simulink model "MMMS_v3"  (R2024b)
settings: Solver=VariableStepAuto  StartTime=0.0  StopTime=60  FixedStep=0.001  RelTol=1e-3
InitFcn:
  | %rho_0t=[0.29;0.29;0.29]; %m
  | %V_0t=[-0.001;-0.001;0];%[-0.0005;-0.0005;0];
  | %w_t=[0;0;-0.002];
  | 
  | 
  | %rho_0t=[0.3;0.3;0.2]; %m
  | %V_0t=[-0.001;-0.001;0];%[-0.0005;-0.0005;0];
  | %w_t=[0;0;-0.001];
values from neighbouring files (symbols this model uses):
  Dt = 0.1    [main_EKF.m]
  Fake_Manip_grad = -0.2.*eye(7)    [Initiate_FQ.m]
  g_cm = zeros(4,4,n)    [Initiate_KUKA_inv.m]    (also in Main_MMMS.m; test_KUKA_elements.m)
  g_It00 = [eye(3) rho_It;0 0 0 1]    [main_EKF.m]
  iota0 = eye(6,6)    [Initiate_KUKA_inv.m]    (also in Main_MMMS.m; test_KUKA_elements.m)
  K_d = 10*[1.3*eye(3) zeros(3);zeros(3) 0.8*eye(3)]    [Initiate_FQ.m]    (also in Initiate_KUKA_inv.m = 5*[0.7*eye(3) zeros(3);zeros(3) 0.5*eye(3)]; MMMS_Initiate_FQ.m; Main_MMMS.m = 5*[0.7*eye(3) zeros(3);zeros(3) 0.5*eye(3)]; test_KUKA_elements.m = 50*[0.7*eye(3) zeros(3);zeros(3) 0.5*eye(3)])
  K_i = 5*[0.1*eye(3) zeros(3);zeros(3) 0.01*eye(3)]    [Initiate_FQ.m]    (also in Initiate_KUKA_inv.m = 5*[0.01*eye(3) zeros(3);zeros(3) 0.001*eye(3)]; MMMS_Initiate_FQ.m; Main_MMMS.m = 5*[0.01*eye(3) zeros(3);zeros(3) 0.001*eye(3)]; test_KUKA_elements.m = 50*[0.01*eye(3) zeros(3);zeros(3) 0.001*eye(3)])
  K_p = 100*[0.1 0 0 0 0 0;0 0.1 0 0 0 0; 0 0 0.1 0 0 0; 0 0 0 0.01 0 0 ... (first row only)    [Initiate_FQ.m]    (also in Initiate_KUKA_inv.m = 5*[0.1 0 0 0 0 0;0 0.1 0 0 0 0; 0 0 0.1 0 0 0; 0 0 0 0.01 0 ; MMMS_Initiate_FQ.m; Main_MMMS.m = 5*[0.1 0 0 0 0 0;0 0.1 0 0 0 0; 0 0 0.1 0 0 0; 0 0 0 0.01 0 ; test_KUKA_elements.m = 50*[0.1 0 0 0 0 0;0 0.1 0 0 0 0; 0 0 0.1 0 0 0; 0 0 0 0.01 0)
  K_w = 200*eye(7)    [Initiate_FQ.m]    (also in MMMS_Initiate_FQ.m)
  K_wd = 2*eye(7)    [Initiate_FQ.m]    (also in MMMS_Initiate_FQ.m)
  m = randn(s,total_time_steps,6)*chol(R)    [main_EKF.m]
  M0 = M_temp.M0.data(:,:,1)    [Initiate_FQ.m]    (also in MMMS_Initiate_FQ.m; test_KUKA_elements.m)
  m0 = robot.Bodies{1,n+1}.Mass    [Initiate_KUKA_inv.m]    (also in Main_MMMS.m; test_KUKA_elements.m)
  m0_frak = diag_M(1:6,1:6)    [Initiate_KUKA_inv.m]    (also in Main_MMMS.m; make_uncertain.m = diag_M_unc(1:6,1:6); test_KUKA_elements.m)
  M0m = M_temp.M0m.data(:,:,1)    [Initiate_FQ.m]    (also in MMMS_Initiate_FQ.m; test_KUKA_elements.m)
  m_diag = diag_M(7:end,7:end)    [Initiate_KUKA_inv.m]    (also in Main_MMMS.m; make_uncertain.m = diag_M_unc(7:end,7:end); test_KUKA_elements.m)
  M_t = (((Adjoint(g_It))'\M_t_body)/(Adjoint(g_It)))    [Initiate_FQ.m]    (also in Initiate_KUKA_inv.m = [eye(3)*mt zeros(3); zeros(3) eye(3)*80]; MMMS_Initiate_FQ.m; Main_MMMS.m = [eye(3)*mt zeros(3); zeros(3) eye(3)*80]; test_KUKA_elements.m = [eye(3)*mt zeros(3); zeros(3) eye(3)*80])
  M_t_body = [eye(3)*mt zeros(3); zeros(3) eye(3)*0.416667]    [Initiate_FQ.m]    (also in MMMS_Initiate_FQ.m)
  mm = zeros(1,n)    [Initiate_KUKA_inv.m]    (also in Main_MMMS.m; test_KUKA_elements.m)
  mu = P0    [Initiate_FQ.m]    (also in Initiate_KUKA_inv.m = zeros(6,1); MMMS_Initiate_FQ.m; Main_MMMS.m = zeros(6,1); make_uncertain.m = P0_unc)
  mu_t = inv((Adjoint(g_It))')*M_t_body*[V_It;w_t]    [Initiate_FQ.m]    (also in Initiate_KUKA_inv.m = M_t*[V_0t;w_t]; MMMS_Initiate_FQ.m; Main_MMMS.m = M_t*[V_0t;w_t]; make_uncertain.m = inv((Adjoint(g_It))')*M_t_body_unc*[V_It;w_t])
  noise_st = 0.000005    (= 5e-06)    [main_EKF.m]
  q_dot_m = [0;0;0;0;0;0;0]    [Initiate_FQ.m]    (also in Initiate_KUKA_inv.m; MMMS_Initiate_FQ.m; Main_MMMS.m; test_KUKA_elements.m = [0])
  q_m = [0.2;1.2;0.3;2.5;0.5;1.5;0.6]    [Initiate_FQ.m]    (also in Initiate_KUKA_inv.m = [0;0;0;0;0;0;0]; MMMS_Initiate_FQ.m = [0.2;0.2;0.3;0.5;0.5;0.5;0.6]; Main_MMMS.m = [0;0;0;0;0;0;0]; test_KUKA_elements.m = [0.2;1.2;0.3;1.8;0.5;1.3;0.6])
  rho_It = [0;0;1.7]    [Initiate_FQ.m]    (also in MMMS_Initiate_FQ.m)
  s = RandStream.create('mrg32k3a','NumStreams',1)    [main_EKF.m]
  sc_size = 1    [Initiate_KUKA_inv.m]    (also in Main_MMMS.m; test_KUKA_elements.m)
  V_It = [0.0005;0.0005;0]    [Initiate_FQ.m]    (also in MMMS_Initiate_FQ.m = [0.001;0.001;0])
  Xi_m_matrix = zeros(6*n,n)    [Initiate_KUKA_inv.m]    (also in Main_MMMS.m)
undefined symbols (not defined in the file or in its folder): g_cm0, I0, Im, Mm, X, Xi_m, Y, Z
libraries: nesl_utility x314, sm_lib x231, robotcorelib x30, simulink x12
(part 10 of 13)

== system MMMS_v3/MMS4/joint//link2/iiwa_link_2 ==
  Inertia : sm_lib/Body Elements/Inertia  InertiaType=Custom  Mass=mm(5)  MassUnits=kg  CenterOfMass=[0, 0, 0]  CenterOfMassUnits=m  MomentsOfInertia=[Im(1,1,5) Im(2,2,5) Im(3,3,5)]  MomentsOfInertiaUnits=kg*m^2  ProductsOfInertia=[Im(3,2,5) Im(3,1,5) Im(2,1,5)]  ProductsOfInertiaUnits=kg*m^2  GraphicType=None  MarkerShape=Inertia  MarkerSize=20  GraphicVisPropType=SimpleVisualProperties  GraphicDiffuseColor=[0.5 0.5 0.5]  GraphicOpacity=1.0  GraphicSpecularColor=[0.5 0.5 0.5 1.0]  GraphicAmbientColor=[0.15 0.15 0.15 1.0]  GraphicEmissiveColor=[0.0 0.0 0.0 1.0]  GraphicShininess=75
  Visual : sm_lib/Body Elements/File Solid  ExtGeomFileName=iiwa_description/meshes/iiwa7/visual/link_2.stl  UnitType=Custom  ExtGeomFileUnits=m  StepReaderType=HEX  ExportConvexHullGeometry=off  InertiaType=Custom  BasedOnType=DensityFromFile  Density=1000  DensityUnits=kg/m^3  Mass=0  MassUnits=kg  CenterOfMass=[0, 0, 0]  CenterOfMassUnits=m  MomentsOfInertia=[0, 0, 0]  MomentsOfInertiaUnits=kg*m^2  ProductsOfInertia=[0, 0, 0]  ProductsOfInertiaUnits=kg*m^2  GraphicType=FromGeometry  MarkerShape=Sphere  MarkerSize=10  GraphicVisPropType=SimpleVisualProperties  GraphicDiffuseColor=[1, 0.423529411765, 0.0392156862745]  GraphicOpacity=1  GraphicSpecularColor=[0.5 0.5 0.5 1.0]  GraphicAmbientColor=[0.15 0.15 0.15 1.0]  GraphicEmissiveColor=[0.0 0.0 0.0 1.0]  GraphicShininess=75  DoExposeReferenceFrame=on  SerializedFrames=<Frames/>
  VisualOriginTransform : sm_lib/Frames and Transforms/Rigid Transform  RotationMethod=RotationSequence  FollAlignAxisA=+X  BaseAlignAxisA=+Y  FollAlignAxisB=+Y  BaseAlignAxisB=+Z  RotationStandardAxis=+Z  RotationAngle=0.0  RotationAngleUnits=deg  RotationArbitraryAxis=[0 0 1]  RotationSequenceAxes=BaseAxes  RotationSequence=XYZ  RotationSequenceAngles=[0, 0, 0]  RotationSequenceAnglesUnits=rad  RotationMatrix=[1 0 0; 0 1 0; 0 0 1]  Quaternion=[1 0 0 0]  TranslationMethod=Cartesian  TranslationCartesianOffset=[0, 0, 0]  TranslationCartesianOffsetUnits=m  TranslationStandardAxis=+Z  TranslationStandardOffset=0  TranslationStandardOffsetUnits=m  TranslationROffset=0  TranslationROffsetUnits=m  TranslationThetaOffset=0  TranslationThetaOffsetUnits=deg  TranslationZOffset=0  TranslationZOffsetUnits=m
  iiwa_joint_3_OriginTransform : sm_lib/Frames and Transforms/Rigid Transform  RotationMethod=RotationMatrix  FollAlignAxisA=+X  BaseAlignAxisA=+Y  FollAlignAxisB=+Y  BaseAlignAxisB=+Z  RotationStandardAxis=+Z  RotationAngle=0.0  RotationAngleUnits=deg  RotationArbitraryAxis=[0 0 1]  RotationSequenceAxes=BaseAxes  RotationSequence=XYZ  RotationSequenceAngles=[1.57079632679, 0, 3.14159265359]  RotationSequenceAnglesUnits=rad  RotationMatrix=g_cm(1:3,1:3,5)  Quaternion=[1 0 0 0]  TranslationMethod=Cartesian  TranslationCartesianOffset=g_cm(1:3,4,5)'  TranslationCartesianOffsetUnits=m  TranslationStandardAxis=+Z  TranslationStandardOffset=0  TranslationStandardOffsetUnits=m  TranslationROffset=0  TranslationROffsetUnits=m  TranslationThetaOffset=0  TranslationThetaOffsetUnits=deg  TranslationZOffset=0  TranslationZOffsetUnits=m
  F : PMIOPort  Side=Left
  F1 : PMIOPort  Port=2  Side=Right
  connections:
  iiwa_joint_3_OriginTransform/LConn1 -- F1/RConn1
  F/RConn1 -- iiwa_joint_3_OriginTransform/RConn1 -- Inertia/RConn1 -- VisualOriginTransform/LConn1
  Visual/RConn1 -- VisualOriginTransform/RConn1

== system MMMS_v3/MMS4/joint//link3/iiwa_link_3 ==
  Inertia : sm_lib/Body Elements/Inertia  InertiaType=Custom  Mass=mm(4)  MassUnits=kg  CenterOfMass=[0, 0, 0]  CenterOfMassUnits=m  MomentsOfInertia=[Im(1,1,4) Im(2,2,4) Im(3,3,4)]  MomentsOfInertiaUnits=kg*m^2  ProductsOfInertia=[Im(3,2,4) Im(3,1,4) Im(2,1,4)]  ProductsOfInertiaUnits=kg*m^2  GraphicType=None  MarkerShape=Inertia  MarkerSize=20  GraphicVisPropType=SimpleVisualProperties  GraphicDiffuseColor=[0.5 0.5 0.5]  GraphicOpacity=1.0  GraphicSpecularColor=[0.5 0.5 0.5 1.0]  GraphicAmbientColor=[0.15 0.15 0.15 1.0]  GraphicEmissiveColor=[0.0 0.0 0.0 1.0]  GraphicShininess=75
  Visual : sm_lib/Body Elements/File Solid  ExtGeomFileName=iiwa_description/meshes/iiwa7/visual/link_3.stl  UnitType=Custom  ExtGeomFileUnits=m  StepReaderType=HEX  ExportConvexHullGeometry=off  InertiaType=Custom  BasedOnType=DensityFromFile  Density=1000  DensityUnits=kg/m^3  Mass=0  MassUnits=kg  CenterOfMass=[0, 0, 0]  CenterOfMassUnits=m  MomentsOfInertia=[0, 0, 0]  MomentsOfInertiaUnits=kg*m^2  ProductsOfInertia=[0, 0, 0]  ProductsOfInertiaUnits=kg*m^2  GraphicType=FromGeometry  MarkerShape=Sphere  MarkerSize=10  GraphicVisPropType=SimpleVisualProperties  GraphicDiffuseColor=[1, 0.423529411765, 0.0392156862745]  GraphicOpacity=1  GraphicSpecularColor=[0.5 0.5 0.5 1.0]  GraphicAmbientColor=[0.15 0.15 0.15 1.0]  GraphicEmissiveColor=[0.0 0.0 0.0 1.0]  GraphicShininess=75  DoExposeReferenceFrame=on  SerializedFrames=<Frames/>
  VisualOriginTransform : sm_lib/Frames and Transforms/Rigid Transform  RotationMethod=RotationSequence  FollAlignAxisA=+X  BaseAlignAxisA=+Y  FollAlignAxisB=+Y  BaseAlignAxisB=+Z  RotationStandardAxis=+Z  RotationAngle=0.0  RotationAngleUnits=deg  RotationArbitraryAxis=[0 0 1]  RotationSequenceAxes=BaseAxes  RotationSequence=XYZ  RotationSequenceAngles=[0, 0, 0]  RotationSequenceAnglesUnits=rad  RotationMatrix=[1 0 0; 0 1 0; 0 0 1]  Quaternion=[1 0 0 0]  TranslationMethod=Cartesian  TranslationCartesianOffset=[0, 0, -0.026]  TranslationCartesianOffsetUnits=m  TranslationStandardAxis=+Z  TranslationStandardOffset=0  TranslationStandardOffsetUnits=m  TranslationROffset=0  TranslationROffsetUnits=m  TranslationThetaOffset=0  TranslationThetaOffsetUnits=deg  TranslationZOffset=0  TranslationZOffsetUnits=m
  iiwa_joint_4_OriginTransform : sm_lib/Frames and Transforms/Rigid Transform  RotationMethod=RotationMatrix  FollAlignAxisA=+X  BaseAlignAxisA=+Y  FollAlignAxisB=+Y  BaseAlignAxisB=+Z  RotationStandardAxis=+Z  RotationAngle=0.0  RotationAngleUnits=deg  RotationArbitraryAxis=[0 0 1]  RotationSequenceAxes=BaseAxes  RotationSequence=XYZ  RotationSequenceAngles=[1.57079632679, 0, 0]  RotationSequenceAnglesUnits=rad  RotationMatrix=g_cm(1:3,1:3,4)  Quaternion=[1 0 0 0]  TranslationMethod=Cartesian  TranslationCartesianOffset=g_cm(1:3,4,4)'  TranslationCartesianOffsetUnits=m  TranslationStandardAxis=+Z  TranslationStandardOffset=0  TranslationStandardOffsetUnits=m  TranslationROffset=0  TranslationROffsetUnits=m  TranslationThetaOffset=0  TranslationThetaOffsetUnits=deg  TranslationZOffset=0  TranslationZOffsetUnits=m
  F : PMIOPort  Side=Left
  F1 : PMIOPort  Port=2  Side=Right
  connections:
  iiwa_joint_4_OriginTransform/LConn1 -- F1/RConn1
  Visual/RConn1 -- VisualOriginTransform/RConn1
  F/RConn1 -- Inertia/RConn1 -- iiwa_joint_4_OriginTransform/RConn1 -- VisualOriginTransform/LConn1

== system MMMS_v3/MMS4/joint//link4/iiwa_link_4 ==
  Inertia : sm_lib/Body Elements/Inertia  InertiaType=Custom  Mass=mm(3)  MassUnits=kg  CenterOfMass=[0, 0, 0]  CenterOfMassUnits=m  MomentsOfInertia=[Im(1,1,3) Im(2,2,3) Im(3,3,3)]  MomentsOfInertiaUnits=kg*m^2  ProductsOfInertia=[Im(3,2,3) Im(3,1,3) Im(2,1,3)]  ProductsOfInertiaUnits=kg*m^2  GraphicType=None  MarkerShape=Inertia  MarkerSize=20  GraphicVisPropType=SimpleVisualProperties  GraphicDiffuseColor=[0.5 0.5 0.5]  GraphicOpacity=1.0  GraphicSpecularColor=[0.5 0.5 0.5 1.0]  GraphicAmbientColor=[0.15 0.15 0.15 1.0]  GraphicEmissiveColor=[0.0 0.0 0.0 1.0]  GraphicShininess=75
  Visual : sm_lib/Body Elements/File Solid  ExtGeomFileName=iiwa_description/meshes/iiwa7/visual/link_4.stl  UnitType=Custom  ExtGeomFileUnits=m  StepReaderType=HEX  ExportConvexHullGeometry=off  InertiaType=Custom  BasedOnType=DensityFromFile  Density=1000  DensityUnits=kg/m^3  Mass=0  MassUnits=kg  CenterOfMass=[0, 0, 0]  CenterOfMassUnits=m  MomentsOfInertia=[0, 0, 0]  MomentsOfInertiaUnits=kg*m^2  ProductsOfInertia=[0, 0, 0]  ProductsOfInertiaUnits=kg*m^2  GraphicType=FromGeometry  MarkerShape=Sphere  MarkerSize=10  GraphicVisPropType=SimpleVisualProperties  GraphicDiffuseColor=[1, 0.423529411765, 0.0392156862745]  GraphicOpacity=1  GraphicSpecularColor=[0.5 0.5 0.5 1.0]  GraphicAmbientColor=[0.15 0.15 0.15 1.0]  GraphicEmissiveColor=[0.0 0.0 0.0 1.0]  GraphicShininess=75  DoExposeReferenceFrame=on  SerializedFrames=<Frames/>
  VisualOriginTransform : sm_lib/Frames and Transforms/Rigid Transform  RotationMethod=RotationSequence  FollAlignAxisA=+X  BaseAlignAxisA=+Y  FollAlignAxisB=+Y  BaseAlignAxisB=+Z  RotationStandardAxis=+Z  RotationAngle=0.0  RotationAngleUnits=deg  RotationArbitraryAxis=[0 0 1]  RotationSequenceAxes=BaseAxes  RotationSequence=XYZ  RotationSequenceAngles=[0, 0, 0]  RotationSequenceAnglesUnits=rad  RotationMatrix=[1 0 0; 0 1 0; 0 0 1]  Quaternion=[1 0 0 0]  TranslationMethod=Cartesian  TranslationCartesianOffset=[0, 0, 0]  TranslationCartesianOffsetUnits=m  TranslationStandardAxis=+Z  TranslationStandardOffset=0  TranslationStandardOffsetUnits=m  TranslationROffset=0  TranslationROffsetUnits=m  TranslationThetaOffset=0  TranslationThetaOffsetUnits=deg  TranslationZOffset=0  TranslationZOffsetUnits=m
  iiwa_joint_5_OriginTransform : sm_lib/Frames and Transforms/Rigid Transform  RotationMethod=RotationMatrix  FollAlignAxisA=+X  BaseAlignAxisA=+Y  FollAlignAxisB=+Y  BaseAlignAxisB=+Z  RotationStandardAxis=+Z  RotationAngle=0.0  RotationAngleUnits=deg  RotationArbitraryAxis=[0 0 1]  RotationSequenceAxes=BaseAxes  RotationSequence=XYZ  RotationSequenceAngles=[-1.57079632679, 3.14159265359, 0]  RotationSequenceAnglesUnits=rad  RotationMatrix=g_cm(1:3,1:3,3)  Quaternion=[1 0 0 0]  TranslationMethod=Cartesian  TranslationCartesianOffset=g_cm(1:3,4,3)'  TranslationCartesianOffsetUnits=m  TranslationStandardAxis=+Z  TranslationStandardOffset=0  TranslationStandardOffsetUnits=m  TranslationROffset=0  TranslationROffsetUnits=m  TranslationThetaOffset=0  TranslationThetaOffsetUnits=deg  TranslationZOffset=0  TranslationZOffsetUnits=m
  F : PMIOPort  Side=Left
  F1 : PMIOPort  Port=2  Side=Right
  connections:
  iiwa_joint_5_OriginTransform/LConn1 -- F1/RConn1
  F/RConn1 -- iiwa_joint_5_OriginTransform/RConn1 -- Inertia/RConn1 -- VisualOriginTransform/LConn1
  Visual/RConn1 -- VisualOriginTransform/RConn1

== system MMMS_v3/MMS4/joint//link5/iiwa_link_5 ==
  Inertia : sm_lib/Body Elements/Inertia  InertiaType=Custom  Mass=mm(2)  MassUnits=kg  CenterOfMass=[0, 0, 0]  CenterOfMassUnits=m  MomentsOfInertia=[Im(1,1,2) Im(2,2,2) Im(3,3,2)]  MomentsOfInertiaUnits=kg*m^2  ProductsOfInertia=[Im(3,2,2) Im(3,1,2) Im(2,1,2)]  ProductsOfInertiaUnits=kg*m^2  GraphicType=None  MarkerShape=Inertia  MarkerSize=20  GraphicVisPropType=SimpleVisualProperties  GraphicDiffuseColor=[0.5 0.5 0.5]  GraphicOpacity=1.0  GraphicSpecularColor=[0.5 0.5 0.5 1.0]  GraphicAmbientColor=[0.15 0.15 0.15 1.0]  GraphicEmissiveColor=[0.0 0.0 0.0 1.0]  GraphicShininess=75
  Visual : sm_lib/Body Elements/File Solid  ExtGeomFileName=iiwa_description/meshes/iiwa7/visual/link_5.stl  UnitType=Custom  ExtGeomFileUnits=m  StepReaderType=HEX  ExportConvexHullGeometry=off  InertiaType=Custom  BasedOnType=DensityFromFile  Density=1000  DensityUnits=kg/m^3  Mass=0  MassUnits=kg  CenterOfMass=[0, 0, 0]  CenterOfMassUnits=m  MomentsOfInertia=[0, 0, 0]  MomentsOfInertiaUnits=kg*m^2  ProductsOfInertia=[0, 0, 0]  ProductsOfInertiaUnits=kg*m^2  GraphicType=FromGeometry  MarkerShape=Sphere  MarkerSize=10  GraphicVisPropType=SimpleVisualProperties  GraphicDiffuseColor=[1, 0.423529411765, 0.0392156862745]  GraphicOpacity=1  GraphicSpecularColor=[0.5 0.5 0.5 1.0]  GraphicAmbientColor=[0.15 0.15 0.15 1.0]  GraphicEmissiveColor=[0.0 0.0 0.0 1.0]  GraphicShininess=75  DoExposeReferenceFrame=on  SerializedFrames=<Frames/>
  VisualOriginTransform : sm_lib/Frames and Transforms/Rigid Transform  RotationMethod=RotationSequence  FollAlignAxisA=+X  BaseAlignAxisA=+Y  FollAlignAxisB=+Y  BaseAlignAxisB=+Z  RotationStandardAxis=+Z  RotationAngle=0.0  RotationAngleUnits=deg  RotationArbitraryAxis=[0 0 1]  RotationSequenceAxes=BaseAxes  RotationSequence=XYZ  RotationSequenceAngles=[0, 0, 0]  RotationSequenceAnglesUnits=rad  RotationMatrix=[1 0 0; 0 1 0; 0 0 1]  Quaternion=[1 0 0 0]  TranslationMethod=Cartesian  TranslationCartesianOffset=[0, 0, -0.026]  TranslationCartesianOffsetUnits=m  TranslationStandardAxis=+Z  TranslationStandardOffset=0  TranslationStandardOffsetUnits=m  TranslationROffset=0  TranslationROffsetUnits=m  TranslationThetaOffset=0  TranslationThetaOffsetUnits=deg  TranslationZOffset=0  TranslationZOffsetUnits=m
  iiwa_joint_6_OriginTransform : sm_lib/Frames and Transforms/Rigid Transform  Commented=on  RotationMethod=RotationSequence  FollAlignAxisA=+X  BaseAlignAxisA=+Y  FollAlignAxisB=+Y  BaseAlignAxisB=+Z  RotationStandardAxis=+Z  RotationAngle=0.0  RotationAngleUnits=deg  RotationArbitraryAxis=[0 0 1]  RotationSequenceAxes=BaseAxes  RotationSequence=XYZ  RotationSequenceAngles=[1.57079632679, 0, 0]  RotationSequenceAnglesUnits=rad  RotationMatrix=[1 0 0; 0 1 0; 0 0 1]  Quaternion=[1 0 0 0]  TranslationMethod=Cartesian  TranslationCartesianOffset=[0, 0.0607 , 0.19]  TranslationCartesianOffsetUnits=m  TranslationStandardAxis=+Z  TranslationStandardOffset=0  TranslationStandardOffsetUnits=m  TranslationROffset=0  TranslationROffsetUnits=m  TranslationThetaOffset=0  TranslationThetaOffsetUnits=deg  TranslationZOffset=0  TranslationZOffsetUnits=m
  iiwa_joint_6_OriginTransform1 : sm_lib/Frames and Transforms/Rigid Transform  RotationMethod=RotationMatrix  FollAlignAxisA=+X  BaseAlignAxisA=+Y  FollAlignAxisB=+Y  BaseAlignAxisB=+Z  RotationStandardAxis=+Z  RotationAngle=0.0  RotationAngleUnits=deg  RotationArbitraryAxis=[0 0 1]  RotationSequenceAxes=BaseAxes  RotationSequence=XYZ  RotationSequenceAngles=[1.57079632679, 0, 0]  RotationSequenceAnglesUnits=rad  RotationMatrix=g_cm(1:3,1:3,2)  Quaternion=[1 0 0 0]  TranslationMethod=Cartesian  TranslationCartesianOffset=g_cm(1:3,4,2)'  TranslationCartesianOffsetUnits=m  TranslationStandardAxis=+Z  TranslationStandardOffset=0  TranslationStandardOffsetUnits=m  TranslationROffset=0  TranslationROffsetUnits=m  TranslationThetaOffset=0  TranslationThetaOffsetUnits=deg  TranslationZOffset=0  TranslationZOffsetUnits=m
  F : PMIOPort  Side=Left
  F1 : PMIOPort  Port=2  Side=Right
  connections:
  iiwa_joint_6_OriginTransform1/LConn1 -- F1/RConn1
  F/RConn1 -- VisualOriginTransform/LConn1 -- Inertia/RConn1 -- iiwa_joint_6_OriginTransform1/RConn1
  Visual/RConn1 -- VisualOriginTransform/RConn1

== system MMMS_v3/MMS4/joint//link6/iiwa_link_6 ==
  Inertia : sm_lib/Body Elements/Inertia  InertiaType=Custom  Mass=mm(1)  MassUnits=kg  CenterOfMass=[0, 0, 0]  CenterOfMassUnits=m  MomentsOfInertia=[Im(1,1,1) Im(2,2,1) Im(3,3,1)]  MomentsOfInertiaUnits=kg*m^2  ProductsOfInertia=[Im(3,2,1) Im(3,1,1) Im(2,1,1)]  ProductsOfInertiaUnits=kg*m^2  GraphicType=None  MarkerShape=Inertia  MarkerSize=20  GraphicVisPropType=SimpleVisualProperties  GraphicDiffuseColor=[0.5 0.5 0.5]  GraphicOpacity=1.0  GraphicSpecularColor=[0.5 0.5 0.5 1.0]  GraphicAmbientColor=[0.15 0.15 0.15 1.0]  GraphicEmissiveColor=[0.0 0.0 0.0 1.0]  GraphicShininess=75
  Visual : sm_lib/Body Elements/File Solid  ExtGeomFileName=iiwa_description/meshes/iiwa7/visual/link_6.stl  UnitType=Custom  ExtGeomFileUnits=m  StepReaderType=HEX  ExportConvexHullGeometry=off  InertiaType=Custom  BasedOnType=DensityFromFile  Density=1000  DensityUnits=kg/m^3  Mass=0  MassUnits=kg  CenterOfMass=[0, 0, 0]  CenterOfMassUnits=m  MomentsOfInertia=[0, 0, 0]  MomentsOfInertiaUnits=kg*m^2  ProductsOfInertia=[0, 0, 0]  ProductsOfInertiaUnits=kg*m^2  GraphicType=FromGeometry  MarkerShape=Sphere  MarkerSize=10  GraphicVisPropType=SimpleVisualProperties  GraphicDiffuseColor=[1, 0.423529411765, 0.0392156862745]  GraphicOpacity=1  GraphicSpecularColor=[0.5 0.5 0.5 1.0]  GraphicAmbientColor=[0.15 0.15 0.15 1.0]  GraphicEmissiveColor=[0.0 0.0 0.0 1.0]  GraphicShininess=75  DoExposeReferenceFrame=on  SerializedFrames=<Frames/>
  VisualOriginTransform : sm_lib/Frames and Transforms/Rigid Transform  RotationMethod=RotationSequence  FollAlignAxisA=+X  BaseAlignAxisA=+Y  FollAlignAxisB=+Y  BaseAlignAxisB=+Z  RotationStandardAxis=+Z  RotationAngle=0.0  RotationAngleUnits=deg  RotationArbitraryAxis=[0 0 1]  RotationSequenceAxes=BaseAxes  RotationSequence=XYZ  RotationSequenceAngles=[0, 0, 0]  RotationSequenceAnglesUnits=rad  RotationMatrix=[1 0 0; 0 1 0; 0 0 1]  Quaternion=[1 0 0 0]  TranslationMethod=Cartesian  TranslationCartesianOffset=[0, 0, 0.0607 ]  TranslationCartesianOffsetUnits=m  TranslationStandardAxis=+Z  TranslationStandardOffset=0  TranslationStandardOffsetUnits=m  TranslationROffset=0  TranslationROffsetUnits=m  TranslationThetaOffset=0  TranslationThetaOffsetUnits=deg  TranslationZOffset=0  TranslationZOffsetUnits=m
  iiwa_joint_7_OriginTransform : sm_lib/Frames and Transforms/Rigid Transform  RotationMethod=RotationMatrix  FollAlignAxisA=+X  BaseAlignAxisA=+Y  FollAlignAxisB=+Y  BaseAlignAxisB=+Z  RotationStandardAxis=+Z  RotationAngle=0.0  RotationAngleUnits=deg  RotationArbitraryAxis=[0 0 1]  RotationSequenceAxes=BaseAxes  RotationSequence=XYZ  RotationSequenceAngles=[-1.57079632679, 3.14159265359, 0]  RotationSequenceAnglesUnits=rad  RotationMatrix=g_cm(1:3,1:3,1)  Quaternion=[1 0 0 0]  TranslationMethod=Cartesian  TranslationCartesianOffset=g_cm(1:3,4,1)'  TranslationCartesianOffsetUnits=m  TranslationStandardAxis=+Z  TranslationStandardOffset=0  TranslationStandardOffsetUnits=m  TranslationROffset=0  TranslationROffsetUnits=m  TranslationThetaOffset=0  TranslationThetaOffsetUnits=deg  TranslationZOffset=0  TranslationZOffsetUnits=m
  F : PMIOPort  Side=Left
  F1 : PMIOPort  Port=2  Side=Right
  connections:
  iiwa_joint_7_OriginTransform/LConn1 -- F1/RConn1
  Visual/RConn1 -- VisualOriginTransform/RConn1
  VisualOriginTransform/LConn1 -- F/RConn1 -- Inertia/RConn1 -- iiwa_joint_7_OriginTransform/RConn1

== system MMMS_v3/MMS4/joint//link7/iiwa_link_7 ==
  Inertia : sm_lib/Body Elements/Inertia  InertiaType=Custom  Mass=m0  MassUnits=kg  CenterOfMass=[0, 0, 0]  CenterOfMassUnits=m  MomentsOfInertia=[I0(1,1) I0(2,2) I0(3,3)]  MomentsOfInertiaUnits=kg*m^2  ProductsOfInertia=[I0(3,2) I0(3,1) I0(2,1)]  ProductsOfInertiaUnits=kg*m^2  GraphicType=None  MarkerShape=Inertia  MarkerSize=20  GraphicVisPropType=SimpleVisualProperties  GraphicDiffuseColor=[0.5 0.5 0.5]  GraphicOpacity=1.0  GraphicSpecularColor=[0.5 0.5 0.5 1.0]  GraphicAmbientColor=[0.15 0.15 0.15 1.0]  GraphicEmissiveColor=[0.0 0.0 0.0 1.0]  GraphicShininess=75
  Visual : sm_lib/Body Elements/File Solid  ExtGeomFileName=iiwa_description/meshes/iiwa7/visual/link_7.stl  UnitType=Custom  ExtGeomFileUnits=m  StepReaderType=HEX  ExportConvexHullGeometry=off  InertiaType=Custom  BasedOnType=DensityFromFile  Density=1000  DensityUnits=kg/m^3  Mass=0  MassUnits=kg  CenterOfMass=[0, 0, 0]  CenterOfMassUnits=m  MomentsOfInertia=[0, 0, 0]  MomentsOfInertiaUnits=kg*m^2  ProductsOfInertia=[0, 0, 0]  ProductsOfInertiaUnits=kg*m^2  GraphicType=FromGeometry  MarkerShape=Sphere  MarkerSize=10  GraphicVisPropType=SimpleVisualProperties  GraphicDiffuseColor=[0.4, 0.4, 0.4]  GraphicOpacity=1  GraphicSpecularColor=[0.5 0.5 0.5 1.0]  GraphicAmbientColor=[0.15 0.15 0.15 1.0]  GraphicEmissiveColor=[0.0 0.0 0.0 1.0]  GraphicShininess=75  DoExposeReferenceFrame=on  SerializedFrames=<Frames/>
  VisualOriginTransform : sm_lib/Frames and Transforms/Rigid Transform  RotationMethod=RotationSequence  FollAlignAxisA=+X  BaseAlignAxisA=+Y  FollAlignAxisB=+Y  BaseAlignAxisB=+Z  RotationStandardAxis=+Z  RotationAngle=0.0  RotationAngleUnits=deg  RotationArbitraryAxis=[0 0 1]  RotationSequenceAxes=BaseAxes  RotationSequence=XYZ  RotationSequenceAngles=[0, 0, 0]  RotationSequenceAnglesUnits=rad  RotationMatrix=[1 0 0; 0 1 0; 0 0 1]  Quaternion=[1 0 0 0]  TranslationMethod=Cartesian  TranslationCartesianOffset=[0, 0, 0]  TranslationCartesianOffsetUnits=m  TranslationStandardAxis=+Z  TranslationStandardOffset=0  TranslationStandardOffsetUnits=m  TranslationROffset=0  TranslationROffsetUnits=m  TranslationThetaOffset=0  TranslationThetaOffsetUnits=deg  TranslationZOffset=0  TranslationZOffsetUnits=m
  iiwa_joint_ee_OriginTransform : sm_lib/Frames and Transforms/Rigid Transform  RotationMethod=RotationMatrix  FollAlignAxisA=+X  BaseAlignAxisA=+Y  FollAlignAxisB=+Y  BaseAlignAxisB=+Z  RotationStandardAxis=+Z  RotationAngle=0.0  RotationAngleUnits=deg  RotationArbitraryAxis=[0 0 1]  RotationSequenceAxes=BaseAxes  RotationSequence=XYZ  RotationSequenceAngles=[0, 0, 0]  RotationSequenceAnglesUnits=rad  RotationMatrix=g_cm0(1:3,1:3)  Quaternion=[1 0 0 0]  TranslationMethod=Cartesian  TranslationCartesianOffset=g_cm0(1:3,4)'  TranslationCartesianOffsetUnits=m  TranslationStandardAxis=+Z  TranslationStandardOffset=0  TranslationStandardOffsetUnits=m  TranslationROffset=0  TranslationROffsetUnits=m  TranslationThetaOffset=0  TranslationThetaOffsetUnits=deg  TranslationZOffset=0  TranslationZOffsetUnits=m
  F : PMIOPort  Side=Left
  F1 : PMIOPort  Port=2  Side=Right
  connections:
  iiwa_joint_ee_OriginTransform/LConn1 -- F1/RConn1
  Visual/RConn1 -- VisualOriginTransform/RConn1
  Inertia/RConn1 -- VisualOriginTransform/LConn1 -- iiwa_joint_ee_OriginTransform/RConn1 -- F/RConn1

== system MMMS_v3/Feedback Transformation/Inverse Dynamics1/C_hat/Lm_partials ==
  q_m : Inport
  Xi_m : Inport  Port=2
  Constant : Constant  Value=iota0
  Lm0partial : MATLAB Function  TreatAsAtomicUnit=on
  Lmpartial : MATLAB Function  TreatAsAtomicUnit=on
  Lm_partial : Outport
  Lm0_partial : Outport  Port=2
  wires:
  Lmpartial/1(Lm_partial) -> Lm_partial/1
  Lm0partial/1(Lm0_partial) -> Lm0_partial/1
  Constant/1 -> Lm0partial/3(iota0), Lmpartial/3(iota0)
  q_m/1 -> Lm0partial/1(q_m), Lmpartial/1(q_m)
  Xi_m/1 -> Lm0partial/2(Xi_m), Lmpartial/2(Xi_m)

== system MMMS_v3/Feedback Transformation/Inverse Dynamics1/C_hat/M_partials ==
  q_m : Inport
  Lm_partial : Inport  Port=2
  Lm0_partial : Inport  Port=3
  Lm : Inport  Port=4
  Lm0 : Inport  Port=5
  V : Inport  Port=6
  " M0partial" : MATLAB Function  TreatAsAtomicUnit=on
  Constant : Constant  Value=iota0
  Constant2 : Constant  Value=Xi_m_matrix
  M0mpartial : MATLAB Function  TreatAsAtomicUnit=on
  Mmpartial : MATLAB Function  TreatAsAtomicUnit=on
  M0_partial : Outport
  M0m_partial : Outport  Port=2
  Mm_partial : Outport  Port=3
  wires:
  Lm_partial/1 -> M0mpartial/8(Lm_partial), Mmpartial/5(Lm_partial)
  q_m/1 -> " M0partial"/1(q_m), M0mpartial/1(q_m), Mmpartial/1(q_m)
  [diag_Mm] -> " M0partial"/5(diag_Mm), M0mpartial/6(diag_Mm), Mmpartial/4(diag_Mm)
  Constant2/1 -> M0mpartial/9(Xi_m_matrix), Mmpartial/2(Xi_m_matrix)
  Lm/1 -> M0mpartial/3(Lm), Mmpartial/3(Lm)
  Mmpartial/1(Mm_partial) -> Mm_partial/1
  M0mpartial/1(M0m_partial) -> M0m_partial/1
  " M0partial"/1(M0_partial) -> M0_partial/1
  Lm0/1 -> M0mpartial/4(Lm0), " M0partial"/2(Lm0)
  Lm0_partial/1 -> " M0partial"/6(Lm0_partial), M0mpartial/7(Lm0_partial)
  Constant/1 -> " M0partial"/4(iota0), M0mpartial/5(iota0)
  V/1 -> M0mpartial/2(V), " M0partial"/3(V)

== system MMMS_v3/Feedback Transformation/Inverse Dynamics1/C_hat1/Lm_partials ==
  q_m : Inport
  Xi_m : Inport  Port=2
  Constant : Constant  Value=iota0
  Lm0partial : MATLAB Function  TreatAsAtomicUnit=on
  Lm0partial_par : MATLAB Function  TreatAsAtomicUnit=on
  Lmpartial : MATLAB Function  TreatAsAtomicUnit=on
  Lmpartial_par : MATLAB Function  TreatAsAtomicUnit=on
  Lm_partial : Outport
  Lm0_partial : Outport  Port=2
  Lm_partial_par : Outport  Port=3
  Lm0_partial_par : Outport  Port=4
  wires:
  Lmpartial/1(Lm_partial) -> Lm_partial/1
  Lm0partial/1(Lm0_partial) -> Lm0_partial/1
  Constant/1 -> Lm0partial_par/3(iota0), Lmpartial_par/3(iota0), Lm0partial/3(iota0), Lmpartial/3(iota0)
  q_m/1 -> Lm0partial_par/1(q_m), Lmpartial_par/1(q_m), Lm0partial/1(q_m), Lmpartial/1(q_m)
  Xi_m/1 -> Lm0partial_par/2(Xi_m), Lmpartial_par/2(Xi_m), Lm0partial/2(Xi_m), Lmpartial/2(Xi_m)
  Lm0partial_par/1(Lm0_partial_par) -> Lm0_partial_par/1
  Lmpartial_par/1(Lm_partial_par) -> Lm_partial_par/1

== system MMMS_v3/Feedback Transformation/Inverse Dynamics1/C_hat1/M_partials ==
  q_m : Inport
  Lm_partial : Inport  Port=2
  Lm0_partial : Inport  Port=3
  Lm : Inport  Port=4
  Lm0 : Inport  Port=5
  Lm_partial_par : Inport  Port=6
  V : Inport  Port=7
  Lm0_partial_par : Inport  Port=8
  " M0partial" : MATLAB Function  TreatAsAtomicUnit=on
  " M0partial_par" : MATLAB Function  TreatAsAtomicUnit=on
  Constant : Constant  Value=iota0
  Constant1 : Constant  Value=Xi_m_matrix
  M0mpartial : MATLAB Function  TreatAsAtomicUnit=on
  M0mpartial_par : MATLAB Function  TreatAsAtomicUnit=on
  Mmpartial : MATLAB Function  TreatAsAtomicUnit=on
  M0_partial : Outport
  M0m_partial : Outport  Port=2
  Mm_partial : Outport  Port=3
  M0m_partial_par : Outport  Port=4
  M0_partial_par : Outport  Port=5
  wires:
  Lm_partial/1 -> M0mpartial_par/8(Lm_partial), M0mpartial/8(Lm_partial), Mmpartial/5(Lm_partial)
  q_m/1 -> M0mpartial_par/1(q_m), " M0partial_par"/1(q_m), Mmpartial/1(q_m), M0mpartial/1(q_m), " M0partial"/1(q_m)
  [diag_Mm] -> M0mpartial_par/6(diag_Mm), " M0partial_par"/5(diag_Mm), " M0partial"/5(diag_Mm), M0mpartial/6(diag_Mm), Mmpartial/4(diag_Mm)
  Constant1/1 -> M0mpartial_par/9(Xi_m_matrix), M0mpartial/9(Xi_m_matrix), Mmpartial/2(Xi_m_matrix)
  Lm/1 -> M0mpartial_par/3(Lm), M0mpartial/3(Lm), Mmpartial/3(Lm)
  Mmpartial/1(Mm_partial) -> Mm_partial/1
  M0mpartial/1(M0m_partial) -> M0m_partial/1
  " M0partial"/1(M0_partial) -> M0_partial/1
  Lm0/1 -> " M0partial"/2(Lm0), M0mpartial_par/4(Lm0), " M0partial_par"/2(Lm0), M0mpartial/4(Lm0)
  Lm0_partial/1 -> " M0partial_par"/6(Lm0_partial), M0mpartial_par/7(Lm0_partial), " M0partial"/6(Lm0_partial), M0mpartial/7(Lm0_partial)
  Constant/1 -> M0mpartial_par/5(iota0), " M0partial_par"/4(iota0), M0mpartial/5(iota0), " M0partial"/4(iota0)
  V/1 -> M0mpartial_par/2(V), " M0partial_par"/3(V), M0mpartial/2(V), " M0partial"/3(V)
  M0mpartial_par/1(M0m_partial_par) -> M0m_partial_par/1
  " M0partial_par"/1(M0_partial_par) -> M0_partial_par/1
  Lm0_partial_par/1 -> " M0partial_par"/7(Lm0_partial_par), M0mpartial_par/10(Lm0_partial_par)
  Lm_partial_par/1 -> M0mpartial_par/11(Lm_partial_par)

== system MMMS_v3/Feedback Transformation1/Inverse Dynamics1/C_hat/Lm_partials ==
  q_m : Inport
  Xi_m : Inport  Port=2
  Constant : Constant  Value=iota0
  Lm0partial : MATLAB Function  TreatAsAtomicUnit=on
  Lmpartial : MATLAB Function  TreatAsAtomicUnit=on
  Lm_partial : Outport
  Lm0_partial : Outport  Port=2
  wires:
  Xi_m/1 -> Lmpartial/2(Xi_m), Lm0partial/2(Xi_m)
  q_m/1 -> Lmpartial/1(q_m), Lm0partial/1(q_m)
  Constant/1 -> Lmpartial/3(iota0), Lm0partial/3(iota0)
  Lm0partial/1(Lm0_partial) -> Lm0_partial/1
  Lmpartial/1(Lm_partial) -> Lm_partial/1

== system MMMS_v3/Feedback Transformation1/Inverse Dynamics1/C_hat/M_partials ==
  q_m : Inport
  Lm_partial : Inport  Port=2
  Lm0_partial : Inport  Port=3
  Lm : Inport  Port=4
  Lm0 : Inport  Port=5
  V : Inport  Port=6
  " M0partial" : MATLAB Function  TreatAsAtomicUnit=on
  Constant : Constant  Value=iota0
  Constant2 : Constant  Value=Xi_m_matrix
  M0mpartial : MATLAB Function  TreatAsAtomicUnit=on
  Mmpartial : MATLAB Function  TreatAsAtomicUnit=on
  M0_partial : Outport
  M0m_partial : Outport  Port=2
  Mm_partial : Outport  Port=3
  wires:
  V/1 -> " M0partial"/3(V), M0mpartial/2(V)
  Constant/1 -> M0mpartial/5(iota0), " M0partial"/4(iota0)
  Lm0_partial/1 -> M0mpartial/7(Lm0_partial), " M0partial"/6(Lm0_partial)
  Lm0/1 -> " M0partial"/2(Lm0), M0mpartial/4(Lm0)
  " M0partial"/1(M0_partial) -> M0_partial/1
  M0mpartial/1(M0m_partial) -> M0m_partial/1
  Mmpartial/1(Mm_partial) -> Mm_partial/1
  Lm/1 -> Mmpartial/3(Lm), M0mpartial/3(Lm)
  Constant2/1 -> Mmpartial/2(Xi_m_matrix), M0mpartial/9(Xi_m_matrix)
  [diag_Mm] -> Mmpartial/4(diag_Mm), M0mpartial/6(diag_Mm), " M0partial"/5(diag_Mm)
  q_m/1 -> Mmpartial/1(q_m), M0mpartial/1(q_m), " M0partial"/1(q_m)
  Lm_partial/1 -> Mmpartial/5(Lm_partial), M0mpartial/8(Lm_partial)

== system MMMS_v3/Feedback Transformation1/Inverse Dynamics1/C_hat1/Lm_partials1 ==
  q_m : Inport
  Xi_m : Inport  Port=2
  Constant : Constant  Value=iota0
  Lm0partial : MATLAB Function  TreatAsAtomicUnit=on
  Lm0partial_par : MATLAB Function  TreatAsAtomicUnit=on
  Lmpartial : MATLAB Function  TreatAsAtomicUnit=on
  Lmpartial_par : MATLAB Function  TreatAsAtomicUnit=on
  Lm_partial : Outport
  Lm0_partial : Outport  Port=2
  Lm_partial_par : Outport  Port=3
  Lm0_partial_par : Outport  Port=4
  wires:
  Lmpartial/1(Lm_partial) -> Lm_partial/1
  Lm0partial/1(Lm0_partial) -> Lm0_partial/1
  Constant/1 -> Lm0partial_par/3(iota0), Lmpartial_par/3(iota0), Lm0partial/3(iota0), Lmpartial/3(iota0)
  q_m/1 -> Lm0partial_par/1(q_m), Lmpartial_par/1(q_m), Lm0partial/1(q_m), Lmpartial/1(q_m)
  Xi_m/1 -> Lm0partial_par/2(Xi_m), Lmpartial_par/2(Xi_m), Lm0partial/2(Xi_m), Lmpartial/2(Xi_m)
  Lm0partial_par/1(Lm0_partial_par) -> Lm0_partial_par/1
  Lmpartial_par/1(Lm_partial_par) -> Lm_partial_par/1

== system MMMS_v3/Feedback Transformation1/Inverse Dynamics1/C_hat1/M_partials1 ==
  q_m : Inport
  Lm_partial : Inport  Port=2
  Lm0_partial : Inport  Port=3
  Lm : Inport  Port=4
  Lm0 : Inport  Port=5
  Lm_partial_par : Inport  Port=6
  V : Inport  Port=7
  Lm0_partial_par : Inport  Port=8
  " M0partial" : MATLAB Function  TreatAsAtomicUnit=on
  " M0partial_par" : MATLAB Function  TreatAsAtomicUnit=on
  Constant : Constant  Value=iota0
  Constant1 : Constant  Value=Xi_m_matrix
  M0mpartial : MATLAB Function  TreatAsAtomicUnit=on
  M0mpartial_par : MATLAB Function  TreatAsAtomicUnit=on
  Mmpartial : MATLAB Function  TreatAsAtomicUnit=on
  M0_partial : Outport
  M0m_partial : Outport  Port=2
  Mm_partial : Outport  Port=3
  M0m_partial_par : Outport  Port=4
  M0_partial_par : Outport  Port=5
  wires:
  Lm_partial/1 -> M0mpartial_par/8(Lm_partial), M0mpartial/8(Lm_partial), Mmpartial/5(Lm_partial)
  q_m/1 -> M0mpartial_par/1(q_m), " M0partial_par"/1(q_m), Mmpartial/1(q_m), M0mpartial/1(q_m), " M0partial"/1(q_m)
  [diag_Mm] -> M0mpartial_par/6(diag_Mm), " M0partial_par"/5(diag_Mm), " M0partial"/5(diag_Mm), M0mpartial/6(diag_Mm), Mmpartial/4(diag_Mm)
  Constant1/1 -> M0mpartial_par/9(Xi_m_matrix), M0mpartial/9(Xi_m_matrix), Mmpartial/2(Xi_m_matrix)
  Lm/1 -> M0mpartial_par/3(Lm), M0mpartial/3(Lm), Mmpartial/3(Lm)
  Mmpartial/1(Mm_partial) -> Mm_partial/1
  M0mpartial/1(M0m_partial) -> M0m_partial/1
  " M0partial"/1(M0_partial) -> M0_partial/1
  Lm0/1 -> " M0partial"/2(Lm0), M0mpartial_par/4(Lm0), " M0partial_par"/2(Lm0), M0mpartial/4(Lm0)
  Lm0_partial/1 -> " M0partial_par"/6(Lm0_partial), M0mpartial_par/7(Lm0_partial), " M0partial"/6(Lm0_partial), M0mpartial/7(Lm0_partial)
  Constant/1 -> M0mpartial_par/5(iota0), " M0partial_par"/4(iota0), M0mpartial/5(iota0), " M0partial"/4(iota0)
  V/1 -> M0mpartial_par/2(V), " M0partial_par"/3(V), M0mpartial/2(V), " M0partial"/3(V)
  M0mpartial_par/1(M0m_partial_par) -> M0m_partial_par/1
  " M0partial_par"/1(M0_partial_par) -> M0_partial_par/1
  Lm0_partial_par/1 -> " M0partial_par"/7(Lm0_partial_par), M0mpartial_par/10(Lm0_partial_par)
  Lm_partial_par/1 -> M0mpartial_par/11(Lm_partial_par)

== system MMMS_v3/Feedback Transformation2/Inverse Dynamics1/C_hat/Lm_partials ==
  q_m : Inport
  Xi_m : Inport  Port=2
  Constant : Constant  Value=iota0
  Lm0partial : MATLAB Function  TreatAsAtomicUnit=on
  Lmpartial : MATLAB Function  TreatAsAtomicUnit=on
  Lm_partial : Outport
  Lm0_partial : Outport  Port=2
  wires:
  Lmpartial/1(Lm_partial) -> Lm_partial/1
  Lm0partial/1(Lm0_partial) -> Lm0_partial/1
  Constant/1 -> Lm0partial/3(iota0), Lmpartial/3(iota0)
  q_m/1 -> Lm0partial/1(q_m), Lmpartial/1(q_m)
  Xi_m/1 -> Lm0partial/2(Xi_m), Lmpartial/2(Xi_m)

== system MMMS_v3/Feedback Transformation2/Inverse Dynamics1/C_hat/M_partials ==
  q_m : Inport
  Lm_partial : Inport  Port=2
  Lm0_partial : Inport  Port=3
  Lm : Inport  Port=4
  Lm0 : Inport  Port=5
  V : Inport  Port=6
  " M0partial" : MATLAB Function  TreatAsAtomicUnit=on
  Constant : Constant  Value=iota0
  Constant2 : Constant  Value=Xi_m_matrix
  M0mpartial : MATLAB Function  TreatAsAtomicUnit=on
  Mmpartial : MATLAB Function  TreatAsAtomicUnit=on
  M0_partial : Outport
  M0m_partial : Outport  Port=2
  Mm_partial : Outport  Port=3
  wires:
  Lm_partial/1 -> M0mpartial/8(Lm_partial), Mmpartial/5(Lm_partial)
  q_m/1 -> " M0partial"/1(q_m), M0mpartial/1(q_m), Mmpartial/1(q_m)
  [diag_Mm] -> " M0partial"/5(diag_Mm), M0mpartial/6(diag_Mm), Mmpartial/4(diag_Mm)
  Constant2/1 -> M0mpartial/9(Xi_m_matrix), Mmpartial/2(Xi_m_matrix)
  Lm/1 -> M0mpartial/3(Lm), Mmpartial/3(Lm)
  Mmpartial/1(Mm_partial) -> Mm_partial/1
  M0mpartial/1(M0m_partial) -> M0m_partial/1
  " M0partial"/1(M0_partial) -> M0_partial/1
  Lm0/1 -> M0mpartial/4(Lm0), " M0partial"/2(Lm0)
  Lm0_partial/1 -> " M0partial"/6(Lm0_partial), M0mpartial/7(Lm0_partial)
  Constant/1 -> " M0partial"/4(iota0), M0mpartial/5(iota0)
  V/1 -> M0mpartial/2(V), " M0partial"/3(V)

== system MMMS_v3/Feedback Transformation2/Inverse Dynamics1/C_hat1/Lm_partials1 ==
  q_m : Inport
  Xi_m : Inport  Port=2
  Constant : Constant  Value=iota0
  Lm0partial : MATLAB Function  TreatAsAtomicUnit=on
  Lm0partial_par : MATLAB Function  TreatAsAtomicUnit=on
  Lmpartial : MATLAB Function  TreatAsAtomicUnit=on
  Lmpartial_par : MATLAB Function  TreatAsAtomicUnit=on
  Lm_partial : Outport
  Lm0_partial : Outport  Port=2
  Lm_partial_par : Outport  Port=3
  Lm0_partial_par : Outport  Port=4
  wires:
  Lmpartial/1(Lm_partial) -> Lm_partial/1
  Lm0partial/1(Lm0_partial) -> Lm0_partial/1
  Constant/1 -> Lm0partial_par/3(iota0), Lmpartial_par/3(iota0), Lm0partial/3(iota0), Lmpartial/3(iota0)
  q_m/1 -> Lm0partial_par/1(q_m), Lmpartial_par/1(q_m), Lm0partial/1(q_m), Lmpartial/1(q_m)
  Xi_m/1 -> Lm0partial_par/2(Xi_m), Lmpartial_par/2(Xi_m), Lm0partial/2(Xi_m), Lmpartial/2(Xi_m)
  Lm0partial_par/1(Lm0_partial_par) -> Lm0_partial_par/1
  Lmpartial_par/1(Lm_partial_par) -> Lm_partial_par/1

== system MMMS_v3/Feedback Transformation2/Inverse Dynamics1/C_hat1/M_partials1 ==
  q_m : Inport
  Lm_partial : Inport  Port=2
  Lm0_partial : Inport  Port=3
  Lm : Inport  Port=4
  Lm0 : Inport  Port=5
  Lm_partial_par : Inport  Port=6
  V : Inport  Port=7
  Lm0_partial_par : Inport  Port=8
  " M0partial" : MATLAB Function  TreatAsAtomicUnit=on
  " M0partial_par" : MATLAB Function  TreatAsAtomicUnit=on
  Constant : Constant  Value=iota0
  Constant1 : Constant  Value=Xi_m_matrix
  M0mpartial : MATLAB Function  TreatAsAtomicUnit=on
  M0mpartial_par : MATLAB Function  TreatAsAtomicUnit=on
  Mmpartial : MATLAB Function  TreatAsAtomicUnit=on
  M0_partial : Outport
  M0m_partial : Outport  Port=2
  Mm_partial : Outport  Port=3
  M0m_partial_par : Outport  Port=4
  M0_partial_par : Outport  Port=5
  wires:
  Lm_partial/1 -> M0mpartial_par/8(Lm_partial), M0mpartial/8(Lm_partial), Mmpartial/5(Lm_partial)
  q_m/1 -> M0mpartial_par/1(q_m), " M0partial_par"/1(q_m), Mmpartial/1(q_m), M0mpartial/1(q_m), " M0partial"/1(q_m)
  [diag_Mm] -> M0mpartial_par/6(diag_Mm), " M0partial_par"/5(diag_Mm), " M0partial"/5(diag_Mm), M0mpartial/6(diag_Mm), Mmpartial/4(diag_Mm)
  Constant1/1 -> M0mpartial_par/9(Xi_m_matrix), M0mpartial/9(Xi_m_matrix), Mmpartial/2(Xi_m_matrix)
  Lm/1 -> M0mpartial_par/3(Lm), M0mpartial/3(Lm), Mmpartial/3(Lm)
  Mmpartial/1(Mm_partial) -> Mm_partial/1
  M0mpartial/1(M0m_partial) -> M0m_partial/1
  " M0partial"/1(M0_partial) -> M0_partial/1
  Lm0/1 -> " M0partial"/2(Lm0), M0mpartial_par/4(Lm0), " M0partial_par"/2(Lm0), M0mpartial/4(Lm0)
  Lm0_partial/1 -> " M0partial_par"/6(Lm0_partial), M0mpartial_par/7(Lm0_partial), " M0partial"/6(Lm0_partial), M0mpartial/7(Lm0_partial)
  Constant/1 -> M0mpartial_par/5(iota0), " M0partial_par"/4(iota0), M0mpartial/5(iota0), " M0partial"/4(iota0)
  V/1 -> M0mpartial_par/2(V), " M0partial_par"/3(V), M0mpartial/2(V), " M0partial"/3(V)
  M0mpartial_par/1(M0m_partial_par) -> M0m_partial_par/1
  " M0partial_par"/1(M0_partial_par) -> M0_partial_par/1
  Lm0_partial_par/1 -> " M0partial_par"/7(Lm0_partial_par), M0mpartial_par/10(Lm0_partial_par)
  Lm_partial_par/1 -> M0mpartial_par/11(Lm_partial_par)

== matlab function MMMS_v3/Inverse Dynamics/C_hat/Lm_partials/Lm0partial ==
  data: q_m input; Lm0_partial output; Xi_m input; iota0 input
function Lm0_partial = Lm0_partial(q_m,Xi_m,iota0)
% Calculates the C_hat_m matrix from base pose and arm joint angles

n=length(q_m);

% Find partial of Lm to joint angles
Lm0_partial=zeros(6*n,6,n); % 6nx6xn
for i=1:n
    for j=1:n
        Lm0_partial(6*(j-1)+1:6*j,1:6,i)=Ad_partial(j,1,i,Xi_m,q_m,iota0); % equation 114 of TRO paper
    end
end

%%%%%%%%%%%%%%%%%%%%%%%%%%%%%%%%%%%%%%%%%%%%%%%%%%%%%%%%%%%%% MUST BE
%%%%%%%%%%%%%%%%%%%%%%%%%%%%%%%%%%%%%%%%%%%%%%%%%%%%%%%%%%%%% CHECKED

== matlab function MMMS_v3/Inverse Dynamics/C_hat/Lm_partials/Lmpartial ==
  data: q_m input; Lm_partial output; Xi_m input; iota0 input
function Lm_partial  = Lm_partial(q_m,Xi_m,iota0)
% Calculates the C_hat_m matrix from base pose and arm joint angles

n=length(q_m);

% Find partial of Lm0 to joint angles
Lm_partial=zeros(6*n,6*n,n); % 6nx6xn
for i=1:n
    Lm_partial(:,:,i)=zeros(6*n,6*n);
    for j=2:n
        for k=2:n
            if j>i && i>=k
                Lm_partial(6*(j-1)+1:6*j,6*(k-2)+1:6*(k-1),i)=Ad_partial(j,k,i,Xi_m,q_m,iota0); % equation 81 of TRO paper
            elseif i==j && i>=k
                Lm_partial(6*(j-1)+1:6*j,6*(k-2)+1:6*(k-1),i)=Ad_partial(j,k,i,Xi_m,q_m,iota0); % equation 81 of TRO paper
            else
                Lm_partial(6*(j-1)+1:6*(j-1)+6,6*(k-2)+1:6*(k-2)+6,i)=zeros(6,6);
            end

        end
    end
end

== matlab function MMMS_v3/Inverse Dynamics/C_hat/M_partials/ M0partial ==
  data: q_m input; M0_partial output; Lm0 input; V input; iota0 input; diag_Mm input; Lm0_partial input
function M0_partial = M0_partial(q_m,Lm0,V,iota0,diag_Mm,Lm0_partial)
% Calculates the C_hat_m matrix from base pose and arm joint angles

n=length(q_m);
b=length(V);

% Find partial of M0 to joint angles
M0_partial=zeros(b,b,n); %initiate
for i=1:n
    temp1=transpose(Lm0_partial(1:end,1:end,i))*diag_Mm*Lm0;
    temp2=transpose(Lm0)*diag_Mm*Lm0_partial(1:end,1:end,i);
    M0_partial(1:b,1:b,i)= iota0'*(temp1+temp2)*iota0; %6x6 %equation 117 of TRO
end

== matlab function MMMS_v3/Inverse Dynamics/C_hat/M_partials/M0mpartial ==
  data: q_m input; M0m_partial output; V input; Lm input; Lm0 input; iota0 input; diag_Mm input; Lm0_partial input; Lm_partial input; Xi_m_matrix input
function M0m_partial = M0m_partial(q_m,V,Lm,Lm0,iota0,diag_Mm,Lm0_partial,Lm_partial, Xi_m_matrix)
% Calculates the C_hat_m matrix from base pose and arm joint angles

n=length(q_m);
b=length(V);

% Find partial of M0m to joint angles
M0m_partial=zeros(b,n,n);
for i=1:n
    temp1=transpose(Lm0_partial(1:end,1:end,i))*diag_Mm*Lm;
    temp2=transpose(Lm0)*diag_Mm*Lm_partial(1:end,1:end,i);
    M0m_partial(1:b,1:n,i)= iota0'*(temp1+temp2)*Xi_m_matrix; % equation 118 of TRO paper
end

== matlab function MMMS_v3/Inverse Dynamics/C_hat/M_partials/Mmpartial ==
  data: q_m input; Mm_partial output; Xi_m_matrix input; Lm input; diag_Mm input; Lm_partial input
function Mm_partial = Mm_partial(q_m,Xi_m_matrix,Lm,diag_Mm,Lm_partial)
% Calculates the C_hat_m matrix from base pose and arm joint angles

n=length(q_m);

% find the non-generalized arm mass matrix'x derivative to joint angles
Mm_partial=zeros(n,n,n);
for i=1:n
    temp=   transpose(Lm_partial(1:6*n,1:6*n,i))*diag_Mm*Lm  +   transpose(Lm)*diag_Mm*Lm_partial(1:6*n,1:6*n,i);
    Mm_partial(1:n,1:n,i)=transpose(Xi_m_matrix)*temp*Xi_m_matrix; %calcualte the derivative of not-augmented arm mass matrix from equation 120 of TRO paper
end

== matlab function MMMS_v3/Inverse Dynamics/C_hat/Mm_hat_partial ==
  data: q_m input; AMA_partial input; Mm_hat_partial output; Mm_partial input
function Mm_hat_partial = Mm_hat_partial(q_m, AMA_partial, Mm_partial)
% Calculates the C_hat_m matrix from base pose and arm joint angles

n=length(q_m);

% find the generalized arm mass matrix'x derivative to joint angles
Mm_hat_partial=zeros(n,n,n);
for i=1:n
    Mm_hat_partial(1:n,1:n,i)=Mm_partial(1:n,1:n,i)-AMA_partial(1:n,1:n,i); %calcualte the derivative of augmented arm mass matrix from equation 119 of TRO paper
end

== matlab function MMMS_v3/Inverse Dynamics/Inverse Dynamics/Ad_g_I0_dot ==
  data: g_I0 input; V_I0 input; Ad_g_I0_dot output
function Ad_g_I0_dot = Ad_g_I0_dot(g_I0,V_I0)
% Calculation of F_mu Eq 30 of paper
Ad_g_I0_dot=adjoint_low(V_I0)'*Adjoint(g_I0)';
% adjoint_low(V_I0)*transpose(Adjoint*(g_I0)))

== matlab function MMMS_v3/Inverse Dynamics/Inverse Dynamics/Ad_g_I0_dot1 ==
  data: V_t input; Ad_g_It_dot output; g_It input
function Ad_g_It_dot = Ad_g_It_dot(V_t,g_It)
% Calculation of F_mu Eq 30 of paper
Ad_g_It_dot=adjoint_low(V_t)'*Adjoint(g_It)';

== matlab function MMMS_v3/Inverse Dynamics/Inverse Dynamics/Ad_g_te_dot ==
  data: V_te input; Ad_g_te_dot output; g_te input
function Ad_g_te_dot = Ad_g_te_dot(V_te,g_te)
% Calculation of F_mu Eq 30 of paper
Ad_g_te_dot=-adjoint_low(V_te)/Adjoint(g_te);

== matlab function MMMS_v3/Inverse Dynamics/Inverse Dynamics/FU ==
  data: MmJcross input; F_U output
function F_U = F_U(MmJcross)
F_U=MmJcross;

== matlab function MMMS_v3/Inverse Dynamics/Inverse Dynamics/Fm ==
  data: MmJcross input; F_m output; A_dot input; Cm_hat input
function F_m = F_m(MmJcross,A_dot,Cm_hat)
% Calculation of F_mu Eq 30 of paper
F_m=MmJcross*(A_dot)+Cm_hat;

== matlab function MMMS_v3/Inverse Dynamics/Inverse Dynamics/Fmu ==
  data: MmJcross input; M0 input; M_0_dot input; g_I0 input; F_mu output; Ad_g_I0_dot input
function F_mu = F_mu(MmJcross,M0,M_0_dot,g_I0,Ad_g_I0_dot)
% Calculation of F_mu Eq 30 of paper
F_mu=-MmJcross*(M0\M_0_dot*inv(M0)*transpose(Adjoint(g_I0))+ ...
    M0\Ad_g_I0_dot);

== matlab function MMMS_v3/Inverse Dynamics/Inverse Dynamics/Inverse Dynamics ==
  data: F_mu output; F_t output; F_m output
function [F_mu,F_t,F_m] = fcn()


% n=length(q_m);

%Calculate Mass Matrix block components
% [ M0m Mm]=Mass_Matrix(q_m,Xi_m);

% A=inverse(M0)*M0m; % Mechanical Connection
% Mm_hat=Mm-transpose(A)*M0*A; %augmented manipulator mass matrix
% V=inverse(M0)*(mu-transpose(A)*q_dot_m); %Spacecraft Velocity

% The augmented Jacobian
% J_aug = J_em-J_e0*A;

% for i=1:n
%     for j=1:n
%         Cm_hat=
%     end
% end 

% Find A_dot thru finding partial of connection A to each joint angle
% A_partial=zeros(6,n,n);
% A_dot=zeros(6,n);
% for i=1:n
%     A_partial(6,n,i)=inverse(M0)*M0_partial(1:6,1:6,i)*inverse(M0)*M0m+inverse(M0)*M0m_partial(6,n,i); % Equation 122
%     A_dot(6,n)=A_dot+A_partial(6,n,i).*q_dot_m(i);
% end


% inverse or moore-penrose inverse of the augmented J2 Jacobian matrix
% if rank(J_aug)==size(J2(1,:))
%     J_inv=inverse(J2);
% else
%     J_inv=pinv(J2);
% end

% MJ_inv=-Mm_hat*J_cross;

% J_em_dot=J_em_dot;
% J_e0_dot=J_e0_dot;

% Form the eventual feedback transformation terms
% F_U=MmJcross; %done
% F_mu=MmJcross*(J_e0_dot*inverse(M0)*transpose(Adjoint*(g_I0))- ...
%     J_e0*inverse(M0)*M_0_dot*inverse(M0)*transpose(Adjoint*(g_I0))+ ...
%     J_e0*inverse(M0)*adjoint_low(inverse(M0*transpose(Adjoint(g_I0))*mu)-A*q_dot_m)); 
% F_t=MmJcross*();
% F_m=MmJcross*(J_em_dot-J_e0_dot*A-J_e0*A_dot)+Cm_hat;

== matlab function MMMS_v3/MMS2/collect positions1 ==
  data: g_ni output; g_n2 input; g_n3 input; g_n4 input; g_n5 input; g_n0 input
function g_ni = collect_poses(g_n2,g_n3,g_n4,g_n5, g_n0)

g_ni=zeros(4,4,4);
% p_joints=zeros(3,5);
g_ni(1,:,:)=g_n2;
g_ni(2,:,:)=g_n3;
g_ni(3,:,:)=g_n4;
g_ni(4,:,:)=g_n5;

== matlab function MMMS_v3/Inverse Dynamics/Inverse Dynamics/MATLAB Function3 ==
  data: MmJcross input; g_te input; F_t output; g_It input; Mt input; Ad_gte_dot input; Ad_gIt_dot input
function F_t = F_t(MmJcross,g_te,g_It,Mt,Ad_gte_dot,Ad_gIt_dot)
% Calculation of F_mu Eq 30 of paper
F_t=-MmJcross*(Ad_gte_dot/Mt*Adjoint(g_It)'+Adjoint(g_te)\(Mt\Ad_gIt_dot));

% F_t=MmJcross*(-adjoint_low(V_te)/Adjoint(g_te)/Adjoint(g_tt)/M_t/Adjoint(g_It)'+...
%     Adjoint()\); 

% J_e0_dot*inverse(M0)*transpose(Adjoint*(g_I0))- ...
%     J_e0*inverse(M0)*M_0_dot*inverse(M0)*transpose(Adjoint*(g_I0))+ ...
%     J_e0*inverse(M0)*adjoint_low(inverse(M0*transpose(Adjoint(g_I0))*mu)-A*q_dot_m)
%     Ad_g_te_dot

== matlab function MMMS_v3/Inverse Dynamics/Inverse Dynamics/MmJcross ==
  data: Mm_hat input; MmJcross output; A input
function MmJcross = MmJcross(Mm_hat, A)

JJ=-A;

A_dagger = ((Mm_hat)\JJ')/((JJ/Mm_hat)*JJ');
MmJcross = Mm_hat*A_dagger;%,10^(-2));

== matlab function MMMS_v3/Inverse Dynamics/Inverse Dynamics/Mm_hat ==
  data: M0 input; Mm_hat output; Mm input; A input
function Mm_hat = Mm_hat(M0,Mm,A)

Mm_hat=Mm-A'*M0*A;

== matlab function MMMS_v3/Feedback Transformation/Inverse Dynamics1/C_hat1/Lm_partials/Lm0partial ==
  data: q_m input; Lm0_partial output; Xi_m input; iota0 input
function Lm0_partial = Lm0_partial(q_m,Xi_m,iota0)
% Calculates the C_hat_m matrix from base pose and arm joint angles

n=length(q_m);

% Find partial of Lm to joint angles
Lm0_partial=zeros(6*n,6,n); % 6nx6xn
for i=1:n
    for j=1:n
        Lm0_partial(6*(j-1)+1:6*j,1:6,i)=Ad_partial(j,1,i,Xi_m,q_m,iota0); % equation 114 of TRO paper
    end
end

%%%%%%%%%%%%%%%%%%%%%%%%%%%%%%%%%%%%%%%%%%%%%%%%%%%%%%%%%%%%% MUST BE
%%%%%%%%%%%%%%%%%%%%%%%%%%%%%%%%%%%%%%%%%%%%%%%%%%%%%%%%%%%%% CHECKED
